simulink model "vRTHS_Compensacion"  (R2021a)
settings: Solver=ode4  StartTime=0.0  StopTime=ttotal  FixedStep=dtsim  RelTol=1e-3
values from neighbouring files (symbols this model uses):
  act_num = act_num(end)    [vRTHS.m]
  adaptivegain = diag(10.^op_location)    [vRTHS.m]
  Derivadas = [u;dudt;dudt2;dudt3]    [vRTHS.m]
  dtsim = 1/fs    (= 0.000244140625)    [vRTHS.m]
  Edificio = ss(ssA,[ssB1 ssB2],ssC,[ssD1 ssD2])    [vRTHS.m]
  max_amb = [amb0max,amb1max,amb2max,amb3max]    [vRTHS.m]
  min_amb = [amb0min,amb1min,amb2min,amb3min]    [vRTHS.m]
  params = parametros    [vRTHS.m]
  sat_limit_lower = -3.8    [vRTHS.m]
  sat_limit_upper = +3.8    (= 3.8)    [vRTHS.m]
  sys_kalman = sys_kalman(4:9,:)    [vRTHS.m]
  tipo_control = 3    [vRTHS.m]
undefined symbols (not defined in the file or in its folder): act_den, denfilter, Kc, numfilter
libraries: simulink x3
settings Model: Creator=cristobal  LastModifiedBy=maryf
settings SolverCC: AlgebraicLoopSolver=TrustRegion
settings DataIOCC: ReturnWorkspaceOutputs=off
settings DebuggingCC: SFMachineParentedDataDiag=warning  ArithmeticOperatorsInVariantConditions=warning
settings SFSimCC: SimUseLocalCustomCode=off  CustomCodeUndefinedFunction=UseInterfaceOnly
settings RTWCC: RTWUseLocalCustomCode=off
settings CodeAppCC: StateflowObjectComments=on

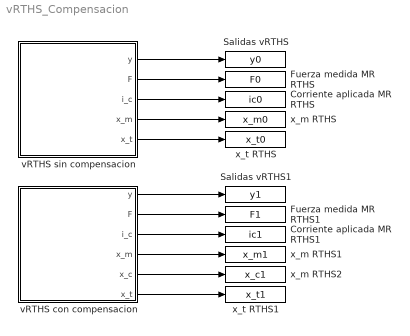
== system vRTHS_Compensacion ==
  Corriente aplicada MR RTHS : ToWorkspace  VariableName=ic0  SaveFormat=Timeseries  SampleTime=-1
  Corriente aplicada MR RTHS1 : ToWorkspace  VariableName=ic1  SaveFormat=Timeseries  SampleTime=-1
  Fuerza medida MR RTHS : ToWorkspace  VariableName=F0  SaveFormat=Timeseries  SampleTime=-1
  Fuerza medida MR RTHS1 : ToWorkspace  VariableName=F1  SaveFormat=Timeseries  SampleTime=-1
  Salidas vRTHS : ToWorkspace  VariableName=y0  SaveFormat=Timeseries  SampleTime=-1
  Salidas vRTHS1 : ToWorkspace  VariableName=y1  SaveFormat=Timeseries  SampleTime=-1
  vRTHS con compensacion : Subsystem
  vRTHS sin compensacion : Subsystem
  x_m RTHS : ToWorkspace  VariableName=x_m0  SaveFormat=Timeseries  SampleTime=-1
  x_m RTHS1 : ToWorkspace  VariableName=x_m1  SaveFormat=Timeseries  SampleTime=-1
  x_m RTHS2 : ToWorkspace  VariableName=x_c1  SaveFormat=Timeseries  SampleTime=-1
  x_t RTHS : ToWorkspace  VariableName=x_t0  SaveFormat=Timeseries  SampleTime=-1
  x_t RTHS1 : ToWorkspace  VariableName=x_t1  SaveFormat=Timeseries  SampleTime=-1
  wires:
  vRTHS sin compensacion/1(y) -> Salidas vRTHS/1
  vRTHS sin compensacion/2(F) -> Fuerza medida MR RTHS/1
  vRTHS sin compensacion/3(i_c) -> Corriente aplicada MR RTHS/1
  vRTHS sin compensacion/4(x_m) -> x_m RTHS/1
  vRTHS sin compensacion/5(x_t) -> x_t RTHS/1
  vRTHS con compensacion/2(F) -> Fuerza medida MR RTHS1/1
  vRTHS con compensacion/1(y) -> Salidas vRTHS1/1
  vRTHS con compensacion/4(x_m) -> x_m RTHS1/1
  vRTHS con compensacion/6(x_t) -> x_t RTHS1/1
  vRTHS con compensacion/3(i_c) -> Corriente aplicada MR RTHS1/1
  vRTHS con compensacion/5(x_c) -> x_m RTHS2/1

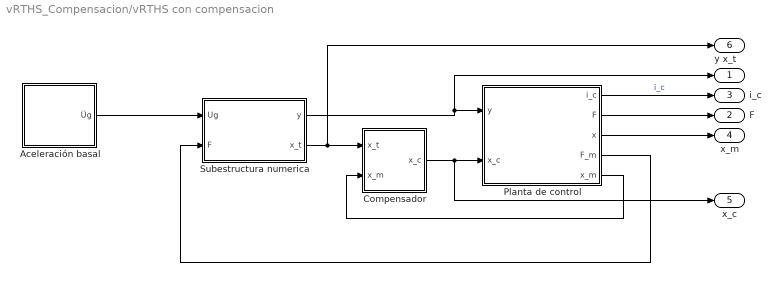
== system vRTHS_Compensacion/vRTHS con compensacion ==
  Aceleración basal : Subsystem
  Compensador : Subsystem
  Planta de control : Subsystem
  Subestructura numerica : Subsystem
  y : Outport  VectorParamsAs1DForOutWhenUnconnected=off
  F : Outport  Port=2  VectorParamsAs1DForOutWhenUnconnected=off
  i_c : Outport  Port=3  VectorParamsAs1DForOutWhenUnconnected=off
  x_m : Outport  Port=4  VectorParamsAs1DForOutWhenUnconnected=off
  x_c : Outport  Port=5  VectorParamsAs1DForOutWhenUnconnected=off
  x_t : Outport  Port=6  VectorParamsAs1DForOutWhenUnconnected=off
  wires:
  Subestructura numerica/1(y) -> y/1, Planta de control/1(y)
  Planta de control/1(i_c) -> i_c/1  "i_c"
  Subestructura numerica/2(x_t) -> Compensador/1(x_t), x_t/1
  Aceleración basal/1(Üg) -> Subestructura numerica/1(Ug)
  Planta de control/4(F_m) -> Subestructura numerica/2("F ")
  Compensador/1(x_c) -> x_c/1, Planta de control/2(x_c)
  Planta de control/5(x_m) -> Compensador/2(x_m)
  Planta de control/2(F) -> F/1
  Planta de control/3(x) -> x_m/1

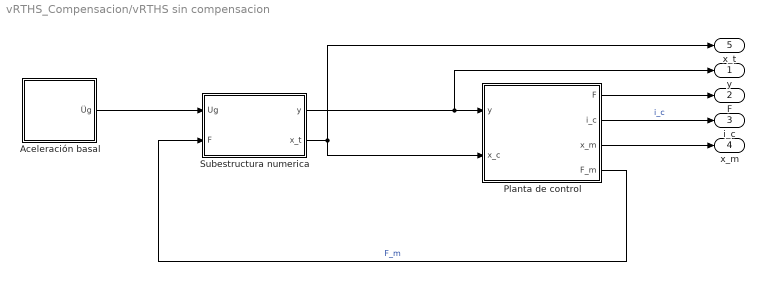
== system vRTHS_Compensacion/vRTHS sin compensacion ==
  Aceleración basal : Subsystem
  Planta de control : Subsystem
  Subestructura numerica : Subsystem
  y : Outport  VectorParamsAs1DForOutWhenUnconnected=off
  F : Outport  Port=2  VectorParamsAs1DForOutWhenUnconnected=off
  i_c : Outport  Port=3  VectorParamsAs1DForOutWhenUnconnected=off
  x_m : Outport  Port=4  VectorParamsAs1DForOutWhenUnconnected=off
  x_t : Outport  Port=5  VectorParamsAs1DForOutWhenUnconnected=off
  wires:
  Subestructura numerica/1(y) -> y/1, Planta de control/1(y)
  Planta de control/2(i_c) -> i_c/1  "i_c"
  Subestructura numerica/2(x_t) -> Planta de control/2(x_c), x_t/1
  Planta de control/3(x_m) -> x_m/1
  Aceleración basal/1(Üg) -> Subestructura numerica/1(Ug)
  Planta de control/4(F_m) -> Subestructura numerica/2("F ")  "F_m"
  Planta de control/1(F) -> F/1

== system vRTHS_Compensacion/vRTHS con compensacion/Aceleración basal ==
  From Workspace1 : FromWorkspace  VariableName=Ug  OutputAfterFinalValue=Setting to zero
  Üg : Outport  VectorParamsAs1DForOutWhenUnconnected=off
  wires:
  From Workspace1/1 -> Üg/1

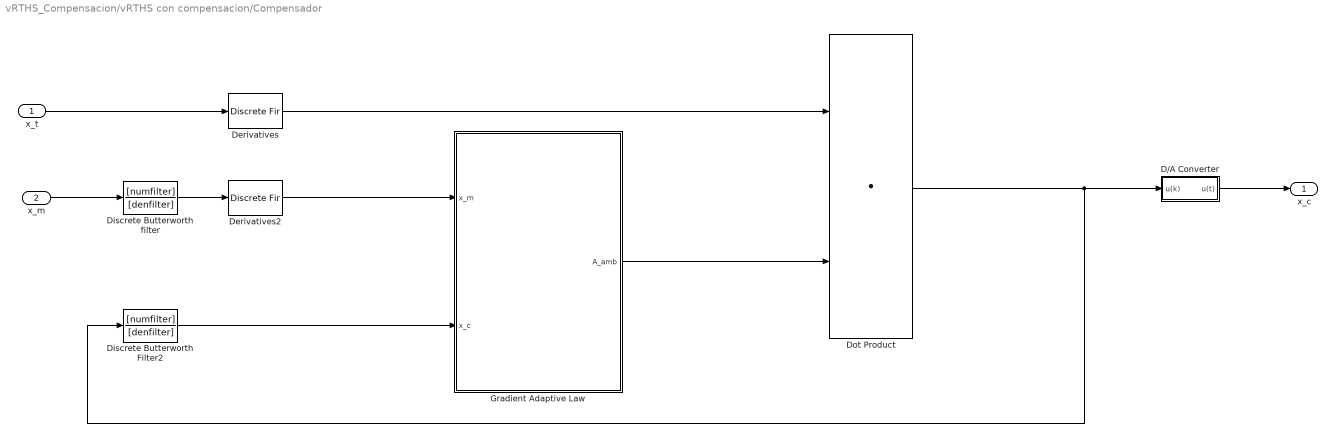
== system vRTHS_Compensacion/vRTHS con compensacion/Compensador ==
  x_t : Inport
  x_m : Inport  Port=2
  D/A Converter : Subsystem
  Derivatives : DiscreteFir  Coefficients=Derivadas
  Derivatives2 : DiscreteFir  Coefficients=Derivadas
  Discrete Butterworth Filter2 : DiscreteTransferFcn  Numerator=[numfilter]  Denominator=[denfilter]
  Discrete Butterworth filter : DiscreteTransferFcn  Numerator=[numfilter]  Denominator=[denfilter]
  Dot Product : DotProduct  InputSameDT=on  OutDataTypeStr=Inherit: Inherit via internal rule
  Gradient Adaptive Law : Subsystem
  x_c : Outport  VectorParamsAs1DForOutWhenUnconnected=off
  wires:
  Derivatives2/1 -> Gradient Adaptive Law/1(x_m)
  Discrete Butterworth Filter2/1 -> Gradient Adaptive Law/2(x_c)
  Discrete Butterworth filter/1 -> Derivatives2/1
  Dot Product/1 -> D/A Converter/1(u(k)), Discrete Butterworth Filter2/1
  Derivatives/1 -> Dot Product/1
  Gradient Adaptive Law/1(A_amb) -> Dot Product/2
  x_t/1 -> Derivatives/1
  x_m/1 -> Discrete Butterworth filter/1
  D/A Converter/1(u(t)) -> x_c/1

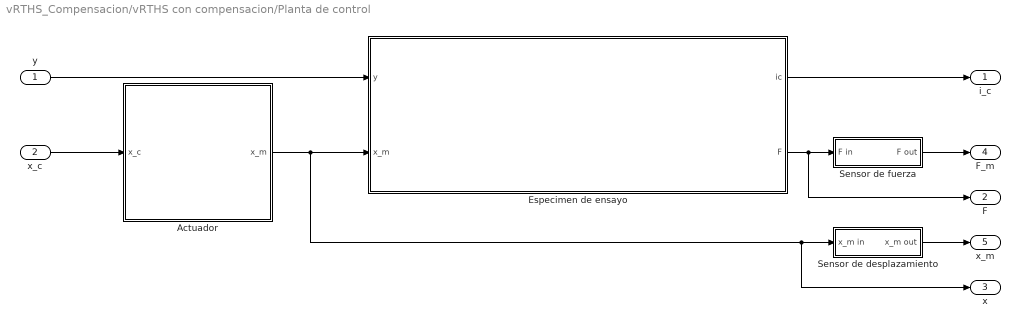
== system vRTHS_Compensacion/vRTHS con compensacion/Planta de control ==
  y : Inport
  x_c : Inport  Port=2
  Actuador : Subsystem
  Especimen de ensayo : Subsystem
  Sensor de desplazamiento : Subsystem
  Sensor de fuerza : Subsystem
  i_c : Outport
  F : Outport  Port=2
  x : Outport  Port=3
  F_m : Outport  Port=4
  x_m : Outport  Port=5
  wires:
  y/1 -> Especimen de ensayo/1(y)
  Especimen de ensayo/1(ic) -> i_c/1
  Actuador/1(x_m) -> x/1, Sensor de desplazamiento/1(x_m in), Especimen de ensayo/2(x_m)
  x_c/1 -> Actuador/1(x_c)
  Sensor de desplazamiento/1(x_m out) -> x_m/1
  Sensor de fuerza/1(F out) -> F_m/1
  Especimen de ensayo/2(F) -> F/1, Sensor de fuerza/1(F in)

== system vRTHS_Compensacion/vRTHS con compensacion/Subestructura numerica ==
  Ug : Inport
  "F " : Inport  Port=2
  Edificio : StateSpace  A=Edificio.A  B=Edificio.B  C=Edificio.C  D=Edificio.D  InitialCondition=0
  Mux : Mux  Inputs=2
  Selector : Selector  InputPortWidth=9  IndexOptions=Index vector (dialog)  Indices=1  OutputSizes=1
  y : Outport
  x_t : Outport  Port=2
  wires:
  Edificio/1 -> Selector/1, y/1  "y"
  Mux/1 -> Edificio/1
  Ug/1 -> Mux/1  "Ug"
  "F "/1 -> Mux/2  "F"
  Selector/1 -> x_t/1

== system vRTHS_Compensacion/vRTHS sin compensacion/Aceleración basal ==
  From Workspace1 : FromWorkspace  VariableName=Ug  OutputAfterFinalValue=Setting to zero
  Üg : Outport  VectorParamsAs1DForOutWhenUnconnected=off
  wires:
  From Workspace1/1 -> Üg/1

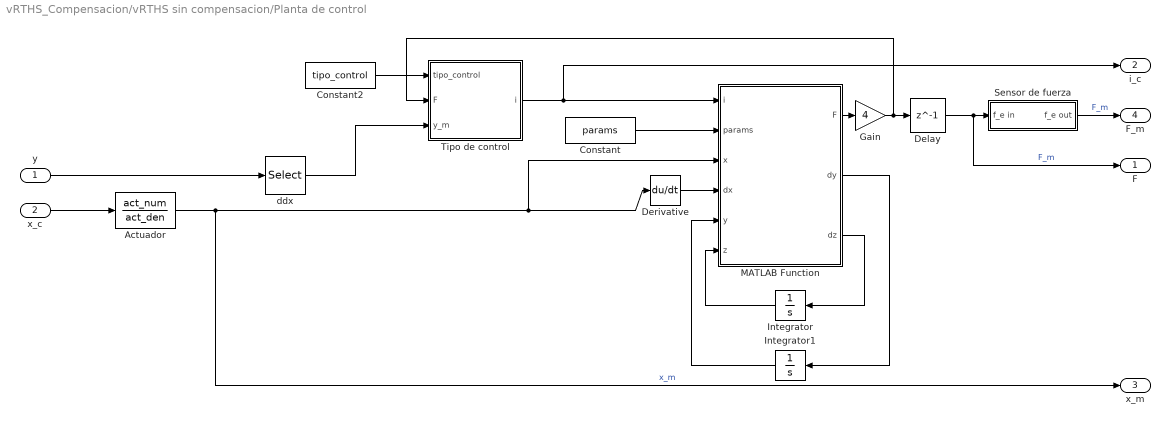
== system vRTHS_Compensacion/vRTHS sin compensacion/Planta de control ==
  y : Inport
  x_c : Inport  Port=2
  Actuador : TransferFcn  Numerator=act_num  Denominator=act_den
  Constant : Constant  Value=params
  Constant2 : Constant  Value=tipo_control
  Delay : Delay  DelayLength=1  InitialCondition=0
  Derivative : Derivative
  Gain : Gain  Gain=4
  Integrator : Integrator
  Integrator1 : Integrator
  MATLAB Function : MATLAB Function  TreatAsAtomicUnit=on
  Sensor de fuerza : Subsystem
  Tipo de control : Subsystem
  ddx : Selector  InputPortWidth=9  IndexOptions=Index vector (dialog)  Indices=7:9  OutputSizes=1
  F : Outport
  i_c : Outport  Port=2
  x_m : Outport  Port=3
  F_m : Outport  Port=4
  wires:
  Integrator1/1 -> MATLAB Function/5(y)
  Constant2/1 -> Tipo de control/1(tipo_control)
  Constant/1 -> MATLAB Function/2(params)
  MATLAB Function/2(dy) -> Integrator1/1
  Tipo de control/1(i) -> i_c/1, MATLAB Function/1(i)
  MATLAB Function/3(dz) -> Integrator/1
  Integrator/1 -> MATLAB Function/6(z)
  y/1 -> ddx/1
  ddx/1 -> Tipo de control/3(y_m)
  x_c/1 -> Actuador/1
  Actuador/1 -> x_m/1, Derivative/1, MATLAB Function/3(x)  "x_m"
  Derivative/1 -> MATLAB Function/4(dx)
  MATLAB Function/1(F) -> Gain/1
  Gain/1 -> Tipo de control/2(F), Delay/1
  Sensor de fuerza/1(f_e out) -> F_m/1  "F_m"
  Delay/1 -> F/1, Sensor de fuerza/1(f_e in)  "F_m"

== system vRTHS_Compensacion/vRTHS sin compensacion/Subestructura numerica ==
  Ug : Inport
  "F " : Inport  Port=2
  Edificio : StateSpace  A=Edificio.A  B=Edificio.B  C=Edificio.C  D=Edificio.D  InitialCondition=0
  Mux : Mux  Inputs=2
  Selector : Selector  InputPortWidth=9  IndexOptions=Index vector (dialog)  Indices=1  OutputSizes=1
  y : Outport
  x_t : Outport  Port=2
  wires:
  Edificio/1 -> Selector/1, y/1  "y"
  Mux/1 -> Edificio/1
  Ug/1 -> Mux/1  "Ug"
  "F "/1 -> Mux/2  "F"
  Selector/1 -> x_t/1

== system vRTHS_Compensacion/vRTHS con compensacion/Compensador/D//A Converter ==
  u(k) : Inport
  Quantizer : Quantizer  QuantizationInterval=quantize_int
  Saturation : Saturate  UpperLimit=sat_limit_upper  LowerLimit=sat_limit_lower
  u(t) : Outport  VectorParamsAs1DForOutWhenUnconnected=off
  wires:
  Saturation/1 -> u(t)/1
  Quantizer/1 -> Saturation/1
  u(k)/1 -> Quantizer/1

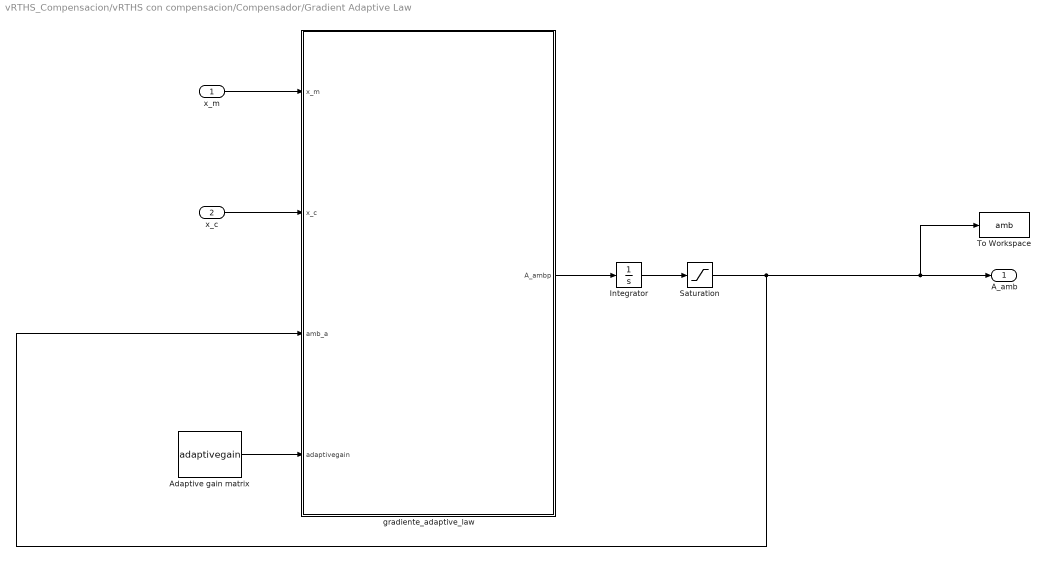
== system vRTHS_Compensacion/vRTHS con compensacion/Compensador/Gradient Adaptive Law ==
  x_m : Inport
  x_c : Inport  Port=2
  Adaptive gain matrix : Constant  Value=adaptivegain
  Integrator : Integrator  InitialCondition=A_amb_i'
  Saturation : Saturate  UpperLimit=[max_amb]  LowerLimit=min_amb
  To Workspace : ToWorkspace  VariableName=amb  SaveFormat=Timeseries  SampleTime=-1
  gradiente_adaptive_law : MATLAB Function  TreatAsAtomicUnit=on
  A_amb : Outport  VectorParamsAs1DForOutWhenUnconnected=off
  wires:
  Integrator/1 -> Saturation/1
  x_c/1 -> gradiente_adaptive_law/2(x_c)
  Adaptive gain matrix/1 -> gradiente_adaptive_law/4(adaptivegain)
  gradiente_adaptive_law/1(A_ambp) -> Integrator/1
  x_m/1 -> gradiente_adaptive_law/1(x_m)
  Saturation/1 -> To Workspace/1, A_amb/1, gradiente_adaptive_law/3(amb_a)

== system vRTHS_Compensacion/vRTHS con compensacion/Planta de control/Actuador ==
  x_c : Inport
  Actuador : TransferFcn  Numerator=act_num  Denominator=act_den
  x_m : Outport
  wires:
  x_c/1 -> Actuador/1
  Actuador/1 -> x_m/1

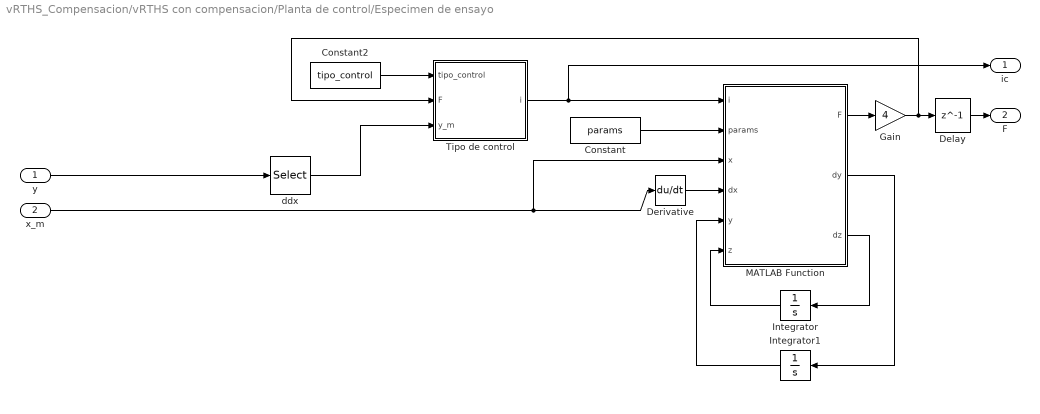
== system vRTHS_Compensacion/vRTHS con compensacion/Planta de control/Especimen de ensayo ==
  y : Inport
  x_m : Inport  Port=2
  Constant : Constant  Value=params
  Constant2 : Constant  Value=tipo_control
  Delay : Delay  DelayLength=1  InitialCondition=0
  Derivative : Derivative
  Gain : Gain  Gain=4
  Integrator : Integrator
  Integrator1 : Integrator
  MATLAB Function : MATLAB Function  TreatAsAtomicUnit=on
  Tipo de control : Subsystem
  ddx : Selector  InputPortWidth=9  IndexOptions=Index vector (dialog)  Indices=7:9  OutputSizes=1
  ic : Outport
  F : Outport  Port=2
  wires:
  Integrator1/1 -> MATLAB Function/5(y)
  Constant2/1 -> Tipo de control/1(tipo_control)
  Tipo de control/1(i) -> ic/1, MATLAB Function/1(i)
  MATLAB Function/2(dy) -> Integrator1/1
  MATLAB Function/3(dz) -> Integrator/1
  MATLAB Function/1(F) -> Gain/1
  ddx/1 -> Tipo de control/3(y_m)
  Integrator/1 -> MATLAB Function/6(z)
  Constant/1 -> MATLAB Function/2(params)
  x_m/1 -> Derivative/1, MATLAB Function/3(x)
  Derivative/1 -> MATLAB Function/4(dx)
  y/1 -> ddx/1
  Delay/1 -> F/1
  Gain/1 -> Tipo de control/2(F), Delay/1

== system vRTHS_Compensacion/vRTHS con compensacion/Planta de control/Sensor de desplazamiento ==
  x_m in : Inport
  Band-Limited White Noise : simulink/Sources/Band-Limited White Noise  Cov=rms_noise_desp  Ts=dtsim  seed=ceil(rand(1)*10000)
  Sum : Sum  Inputs=|++
  Unit Delay : UnitDelay  SampleTime=-1  HasFrameUpgradeWarning=on
  x_m out : Outport  VectorParamsAs1DForOutWhenUnconnected=off
  wires:
  Band-Limited White Noise/1 -> Sum/2
  Sum/1 -> Unit Delay/1
  x_m in/1 -> Sum/1
  Unit Delay/1 -> x_m out/1

== system vRTHS_Compensacion/vRTHS con compensacion/Planta de control/Sensor de fuerza ==
  F in : Inport
  Band-Limited White Noise : simulink/Sources/Band-Limited White Noise  Cov=rms_noise_F  Ts=dtsim  seed=ceil(rand(1)*100)
  Sum : Sum  Inputs=|++
  Unit Delay : UnitDelay  SampleTime=-1  HasFrameUpgradeWarning=on
  F out : Outport  VectorParamsAs1DForOutWhenUnconnected=off
  wires:
  F in/1 -> Sum/1
  Sum/1 -> Unit Delay/1
  Band-Limited White Noise/1 -> Sum/2
  Unit Delay/1 -> F out/1

== system vRTHS_Compensacion/vRTHS sin compensacion/Planta de control/Sensor de fuerza ==
  f_e in : Inport
  Band-Limited White Noise : simulink/Sources/Band-Limited White Noise  Cov=rms_noise_F  Ts=dtsim  seed=ceil(rand(1)*100)
  Sum : Sum  Inputs=|++
  Unit Delay : UnitDelay  SampleTime=-1  HasFrameUpgradeWarning=on
  f_e out : Outport  VectorParamsAs1DForOutWhenUnconnected=off
  wires:
  f_e in/1 -> Sum/1
  Sum/1 -> Unit Delay/1
  Band-Limited White Noise/1 -> Sum/2
  Unit Delay/1 -> f_e out/1

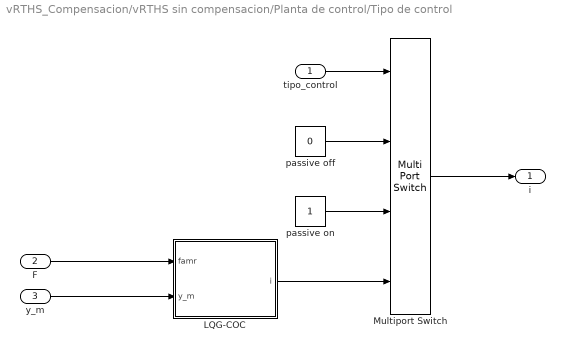
== system vRTHS_Compensacion/vRTHS sin compensacion/Planta de control/Tipo de control ==
  tipo_control : Inport
  F : Inport  Port=2
  y_m : Inport  Port=3
  LQG-COC : Subsystem
  Multiport Switch : MultiPortSwitch
  passive off : Constant  Value=0
  passive on : Constant
  i : Outport
  wires:
  tipo_control/1 -> Multiport Switch/1
  Multiport Switch/1 -> i/1
  passive off/1 -> Multiport Switch/2
  passive on/1 -> Multiport Switch/3
  LQG-COC/1(i) -> Multiport Switch/4
  y_m/1 -> LQG-COC/2(y_m)
  F/1 -> LQG-COC/1(famr)

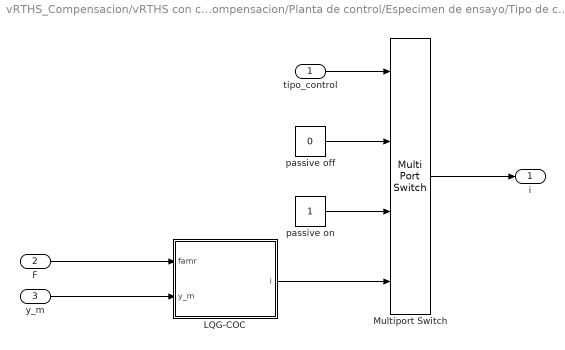
== system vRTHS_Compensacion/vRTHS con compensacion/Planta de control/Especimen de ensayo/Tipo de control ==
  tipo_control : Inport
  F : Inport  Port=2
  y_m : Inport  Port=3
  LQG-COC : Subsystem
  Multiport Switch : MultiPortSwitch
  passive off : Constant  Value=0
  passive on : Constant
  i : Outport
  wires:
  tipo_control/1 -> Multiport Switch/1
  Multiport Switch/1 -> i/1
  passive off/1 -> Multiport Switch/2
  passive on/1 -> Multiport Switch/3
  LQG-COC/1(i) -> Multiport Switch/4
  y_m/1 -> LQG-COC/2(y_m)
  F/1 -> LQG-COC/1(famr)

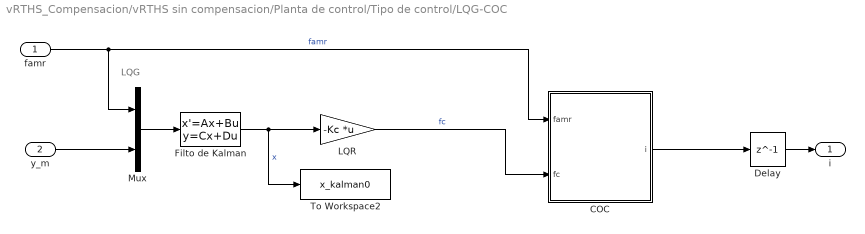
== system vRTHS_Compensacion/vRTHS sin compensacion/Planta de control/Tipo de control/LQG-COC ==
  note: LQG
  famr : Inport
  y_m : Inport  Port=2
  COC : MATLAB Function  TreatAsAtomicUnit=on
  Delay : Delay  DelayLength=1  InitialCondition=0
  Filto de Kalman : StateSpace  A=sys_kalman.a  B=sys_kalman.b  C=sys_kalman.c  D=sys_kalman.d  InitialCondition=0
  LQR : Gain  Gain=-Kc  Multiplication=Matrix(K*u) (u vector)
  Mux : Mux  Inputs=2
  To Workspace2 : ToWorkspace  VariableName=x_kalman0  SaveFormat=Timeseries  SampleTime=-1
  i : Outport
  wires:
  Mux/1 -> Filto de Kalman/1
  famr/1 -> COC/1(famr), Mux/1  "famr"
  y_m/1 -> Mux/2
  Filto de Kalman/1 -> To Workspace2/1, LQR/1  "x"
  Delay/1 -> i/1
  COC/1(i) -> Delay/1
  LQR/1 -> COC/2(fc)  "fc"

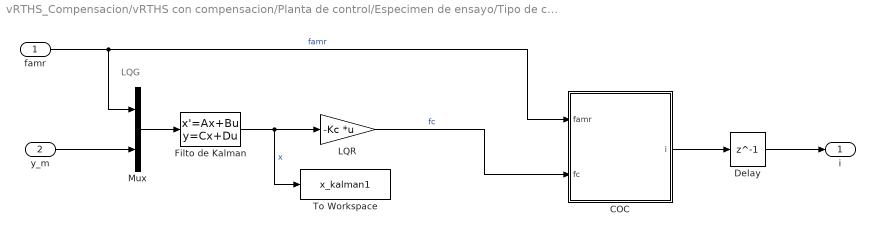
== system vRTHS_Compensacion/vRTHS con compensacion/Planta de control/Especimen de ensayo/Tipo de control/LQG-COC ==
  note: LQG
  famr : Inport
  y_m : Inport  Port=2
  COC : MATLAB Function  TreatAsAtomicUnit=on
  Delay : Delay  DelayLength=1  InitialCondition=0
  Filto de Kalman : StateSpace  A=sys_kalman.a  B=sys_kalman.b  C=sys_kalman.c  D=sys_kalman.d  InitialCondition=0
  LQR : Gain  Gain=-Kc  Multiplication=Matrix(K*u) (u vector)
  Mux : Mux  Inputs=2
  To Workspace : ToWorkspace  VariableName=x_kalman1  SaveFormat=Timeseries  SampleTime=-1
  i : Outport
  wires:
  Mux/1 -> Filto de Kalman/1
  famr/1 -> COC/1(famr), Mux/1  "famr"
  y_m/1 -> Mux/2
  Filto de Kalman/1 -> To Workspace/1, LQR/1  "x"
  Delay/1 -> i/1
  COC/1(i) -> Delay/1
  LQR/1 -> COC/2(fc)  "fc"

== matlab function vRTHS_Compensacion/vRTHS sin compensacion/Planta de control/MATLAB Function ==
  data: i input; params input; x input; dx input; y input; z input; F output size=1; dy output; dz output
function [F,dy,dz] = fcn(i,params,x,dx,y,z)
    A = 300;   
    n = 2;   
    k0 = params(1);
    k1 = params(2);
    x0 = params(3);
    alpha = params(4)*i^2+params(5)*i+params(6);
    gamma = params(7)*exp(params(8)*i);
    beta = gamma;
    c0 = params(9)*i+params(10);
    c1 = params(11)*i+params(12);

    x = x*1000; % el modelo está en mm N
    dx = dx*1000;
    dy = 1/(c0+c1)*(alpha*z+k0*(x-y)+c0*dx);
    dz = -gamma*abs(dx-dy)*((abs(z))^(n-1))*z-beta*(dx-dy)*(abs(z)^n)+A*(dx-dy);
    F  = c1*dy+k1*(x-x0);

== matlab function vRTHS_Compensacion/vRTHS con compensacion/Planta de control/Especimen de ensayo/MATLAB Function ==
  data: i input; params input; x input; dx input; y input; z input; F output size=1; dy output; dz output
function [F,dy,dz] = fcn(i,params,x,dx,y,z)
    A = 300;   
    n = 2;   
    k0 = params(1);
    k1 = params(2);
    x0 = params(3);
    alpha = params(4)*i^2+params(5)*i+params(6);
    gamma = params(7)*exp(params(8)*i);
    beta = gamma;
    c0 = params(9)*i+params(10);
    c1 = params(11)*i+params(12);

    x = x*1000; % el modelo está en mm N
    dx = dx*1000;
    dy = 1/(c0+c1)*(alpha*z+k0*(x-y)+c0*dx);
    dz = -gamma*abs(dx-dy)*((abs(z))^(n-1))*z-beta*(dx-dy)*(abs(z)^n)+A*(dx-dy);
    F  = c1*dy+k1*(x-x0);

== matlab function vRTHS_Compensacion/vRTHS con compensacion/Compensador/Gradient Adaptive Law/gradiente_adaptive_law ==
  data: x_m input; x_c input; amb_a input; A_ambp output; adaptivegain input
function A_ambp   = fcn(x_m,x_c,amb_a,adaptivegain)
error=(x_c-amb_a'*x_m)/(1+(x_m'*x_m));
A_ambp=adaptivegain*error*x_m;

== matlab function vRTHS_Compensacion/vRTHS sin compensacion/Planta de control/Tipo de control/LQG-COC/COC ==
  data: famr input; i output; fc input
function i = fcn(famr,fc)
if abs(fc)>abs(famr)
    i = 1;
else
    i = 0;
end

== matlab function vRTHS_Compensacion/vRTHS con compensacion/Planta de control/Especimen de ensayo/Tipo de control/LQG-COC/COC ==
  data: famr input; i output; fc input
function i = fcn(famr,fc)
if abs(fc)>abs(famr)
    i = 1;
else
    i = 0;
end
